simulink model "Model"  (R2023b)
settings: Solver=VariableStepAuto  StartTime=0.0  StopTime=1  RelTol=1e-3
values from neighbouring files (symbols this model uses):
  BEES = 10    [HEMS_Parameters.m]
settings Model: Creator=jussi  LastModifiedBy=jussi
settings GRTTargetCC: LogVarNameModifier=none

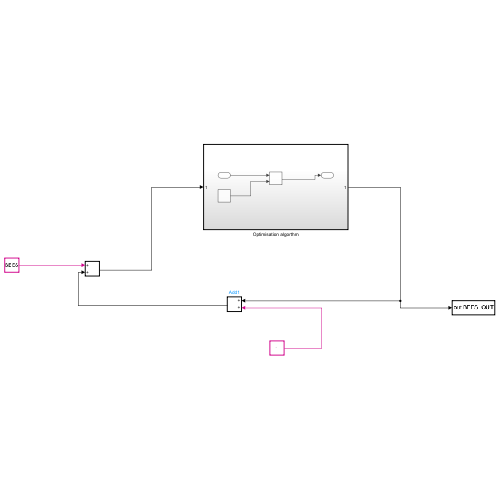
[thumbnail: Simulink's stored preview of the top-level diagram]
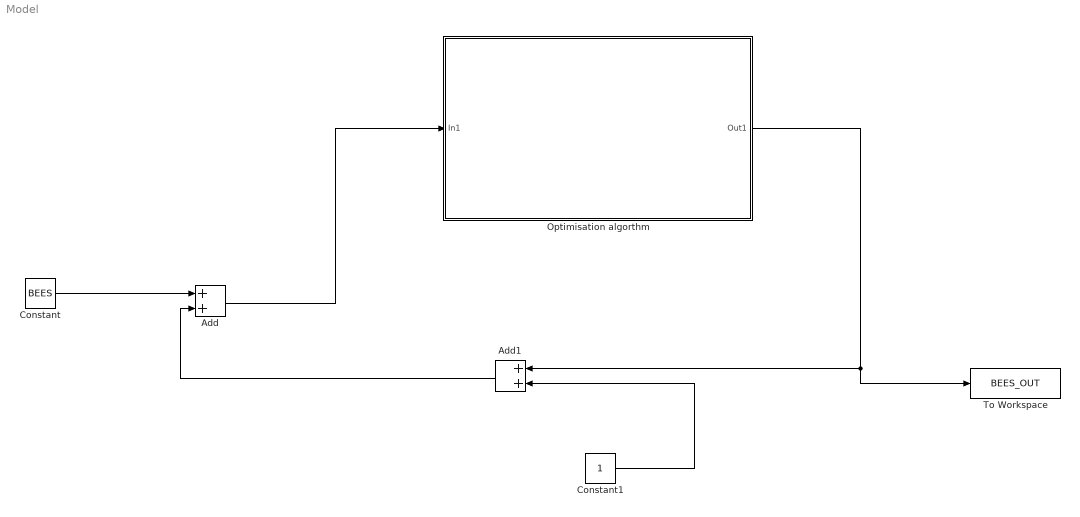
== system Model ==
  Add : Sum
  Add1 : Sum
  Constant : Constant  Value=BEES
  Constant1 : Constant
  Optimisation algorthm : Subsystem
  To Workspace : ToWorkspace  VariableName=BEES_OUT  SaveFormat=Timeseries  SampleTime=-1
  wires:
  Optimisation algorthm/1(Out1) -> To Workspace/1, Add1/1
  Add/1 -> Optimisation algorthm/1(In1)
  Constant/1 -> Add/1
  Constant1/1 -> Add1/2
  Add1/1 -> Add/2

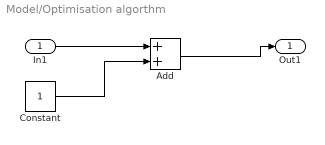
== system Model/Optimisation algorthm ==
  In1 : Inport
  Add : Sum
  Constant : Constant
  Out1 : Outport
  wires:
  In1/1 -> Add/1
  Add/1 -> Out1/1
  Constant/1 -> Add/2
